simulink model "fahrenheitTo_celsiue"  (R2024b)
settings: Solver=VariableStepAuto  StartTime=0.0  StopTime=10  RelTol=1e-3
values from neighbouring files (symbols this model uses):
  C = input(promt)    [scriptFor_fahrenheitTo_celsiue.m]
settings Model: Creator=admin  LastModifiedBy=admin

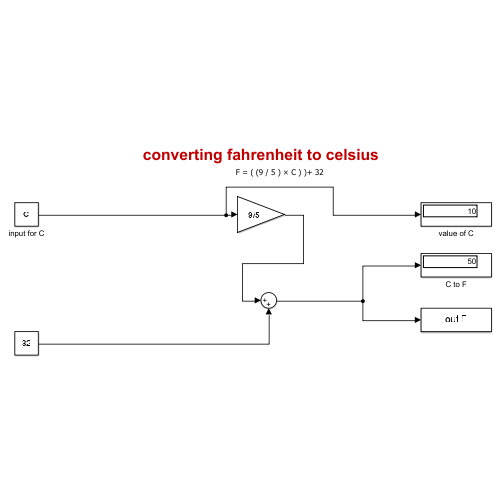
[thumbnail: Simulink's stored preview of the top-level diagram]
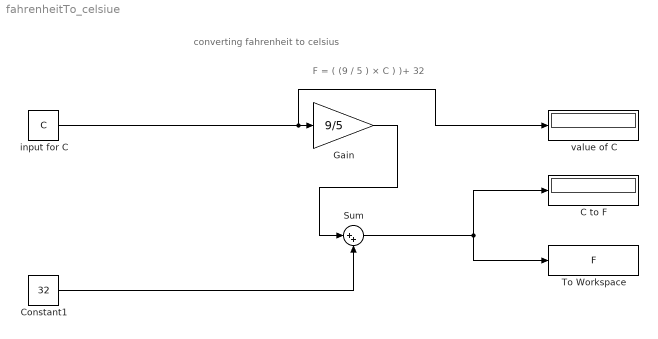
== system fahrenheitTo_celsiue ==
  note: F = ( (9 / 5 )​ × C ) )+ 32
  note: converting fahrenheit to celsius
  C to F : Display
  Constant1 : Constant  Value=32
  Gain : Gain  Gain=9/5
  Sum : Sum  Inputs=|++
  To Workspace : ToWorkspace  VariableName=F  SaveFormat=Timeseries  SampleTime=-1
  input for C : Constant  Value=C
  value of C : Display
  wires:
  input for C/1 -> value of C/1, Gain/1
  Gain/1 -> Sum/1
  Constant1/1 -> Sum/2
  Sum/1 -> To Workspace/1, C to F/1
